simulink library "lat_dyn_haul_00"  (R2025a)
settings: Solver=VariableStepAuto  StartTime=0.0  StopTime=10.0  RelTol=1e-3
settings Model: Creator=marti343  LastModifiedBy=marti343

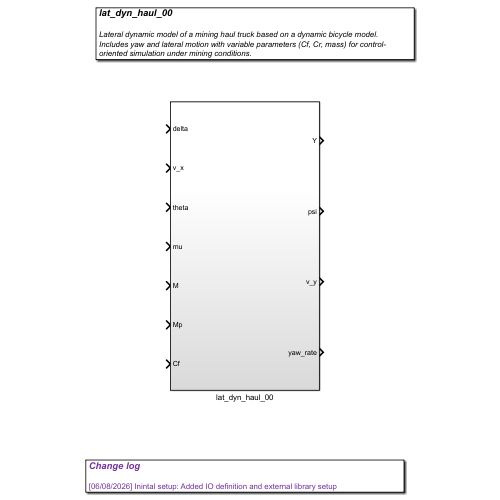
[thumbnail: Simulink's stored preview of the top-level diagram]
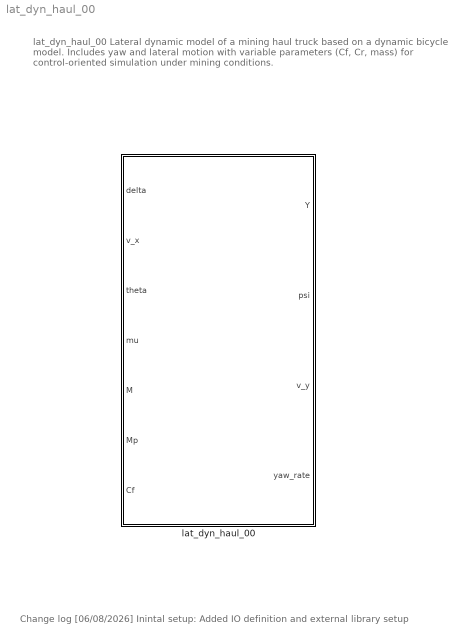
== system lat_dyn_haul_00 ==
  note: lat_dyn_haul_00
      |
      | Lateral dynamic model of a mining haul truck based on a dynamic bicycle model.
      | Includes yaw and lateral motion with variable parameters (Cf, Cr, mass) for control-oriented simulation under mining conditions.
  note: Change log
      |
      | [06/08/2026] Inintal setup: Added IO definition and external library setup
  lat_dyn_haul_00 : Subsystem

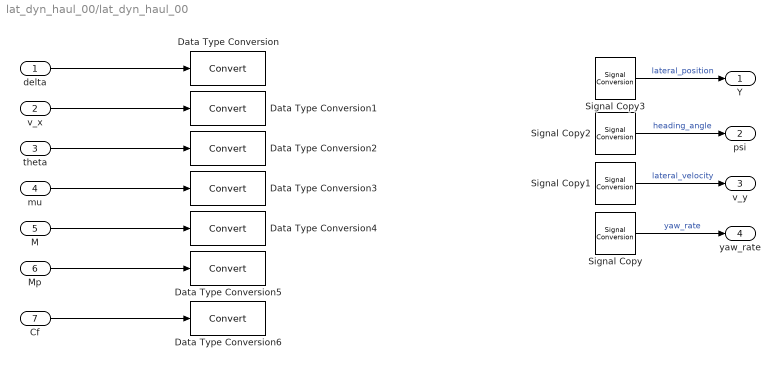
== system lat_dyn_haul_00/lat_dyn_haul_00 ==
  delta : Inport
  v_x : Inport  Port=2
  theta : Inport  Port=3
  mu : Inport  Port=4
  M : Inport  Port=5
  Mp : Inport  Port=6
  Cf : Inport  Port=7
  Data Type Conversion{,1..6} (7 alike) : DataTypeConversion  SaturateOnIntegerOverflow=off  RndMeth=Floor
  Signal Copy{,1..3} (4 alike) : SignalConversion  OverrideOpt=off
  Y : Outport
  psi : Outport  Port=2
  v_y : Outport  Port=3
  yaw_rate : Outport  Port=4
  wires:
  delta/1 -> Data Type Conversion/1
  M/1 -> Data Type Conversion4/1
  Cf/1 -> Data Type Conversion6/1
  Signal Copy2/1 -> psi/1  "heading_angle"
  mu/1 -> Data Type Conversion3/1
  theta/1 -> Data Type Conversion2/1
  Mp/1 -> Data Type Conversion5/1
  Signal Copy3/1 -> Y/1  "lateral_position"
  v_x/1 -> Data Type Conversion1/1
  Signal Copy/1 -> yaw_rate/1  "yaw_rate"
  Signal Copy1/1 -> v_y/1  "lateral_velocity"
